simulink model "MPSLab4ES"  (R2014b)
settings: Solver=ode3  StartTime=0.0  StopTime=10.0  FixedStep=0.01  RelTol=1e-3
settings Model: Creator=kiril_000  LastModifiedBy=kiril_000

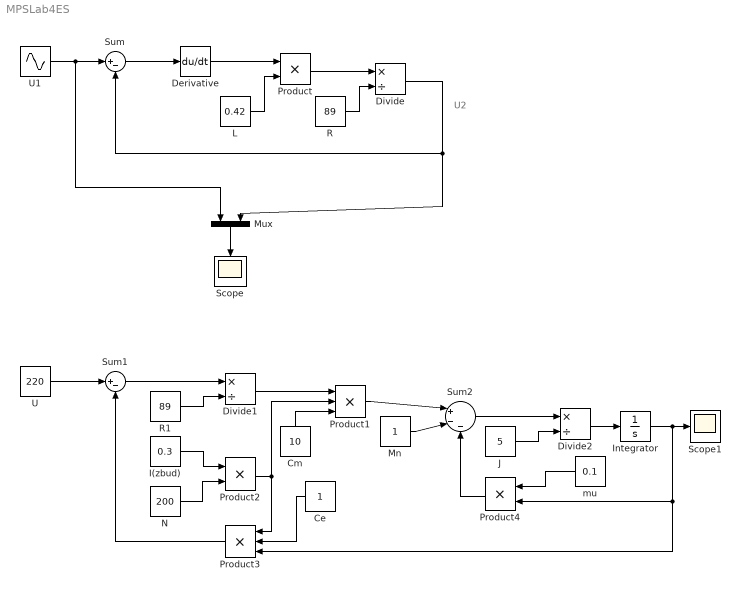
== system MPSLab4ES ==
  note: U2
  Ce : Constant
  Cm : Constant  Value=10
  Derivative : Derivative
  Divide : Product  Inputs=*/
  Divide1 : Product  Inputs=*/
  Divide2 : Product  Inputs=*/
  I(zbud) : Constant  Value=0.3
  Integrator : Integrator
  J : Constant  Value=5
  L : Constant  Value=0.42
  Mn : Constant
  Mux : Mux  Inputs=2
  N : Constant  Value=200
  Product : Product
  Product1 : Product  Inputs=3
  Product2 : Product
  Product3 : Product  Inputs=3
  Product4 : Product
  R : Constant  Value=89
  R1 : Constant  Value=89
  Scope : Scope
  Scope1 : Scope
  Sum : Sum  Inputs=|+-
  Sum1 : Sum  Inputs=|+-
  Sum2 : Sum  Inputs=|+--
  U : Constant  Value=220
  U1 : Sin  Frequency=3  SampleTime=0
  mu : Constant  Value=0.1
  wires:
  U1/1 -> Mux/1, Sum/1
  Sum/1 -> Derivative/1
  Derivative/1 -> Product/1
  L/1 -> Product/2
  Product/1 -> Divide/1
  R/1 -> Divide/2
  Divide/1 -> Mux/2, Sum/2
  Mux/1 -> Scope/1
  U/1 -> Sum1/1
  Sum1/1 -> Divide1/1
  Divide1/1 -> Product1/1
  Product1/1 -> Sum2/1
  Mn/1 -> Sum2/2
  Sum2/1 -> Divide2/1
  J/1 -> Divide2/2
  Divide2/1 -> Integrator/1
  Integrator/1 -> Product3/3, Product4/2, Scope1/1
  Cm/1 -> Product1/3
  R1/1 -> Divide1/2
  I(zbud)/1 -> Product2/1
  N/1 -> Product2/2
  Product2/1 -> Product3/1, Product1/2
  Product3/1 -> Sum1/2
  Ce/1 -> Product3/2
  Product4/1 -> Sum2/3
  mu/1 -> Product4/1
